simulink library "THB_fixed_mdot"  (Simulink 8.2)
settings: Solver=ode45  StartTime=0.0  StopTime=10.0  RelTol=1e-3
libraries: carnot x1
settings Model: Creator=lena.frank  LastModifiedBy=awohlfei

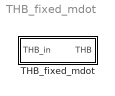
== system THB_fixed_mdot ==
  THB_fixed_mdot : Subsystem  InitFcn=load('THB.mat');  mask(set masssflow in THB){m=10/60}
      mask prompts: m "massflow in kg/s"
      mask help: Set a constant massflow in the thermo-hydraulic vector.

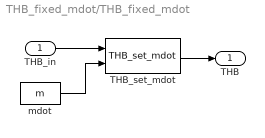
== system THB_fixed_mdot/THB_fixed_mdot ==
  THB_in : Inport
  THB_set_mdot : carnot/Source/Simple/THB_set_mdot
  mdot : Constant  Value=m
  THB : Outport
  wires:
  THB_set_mdot/1 -> THB/1
  THB_in/1 -> THB_set_mdot/1
  mdot/1 -> THB_set_mdot/2
